simulink model "Quadcopter_v2_full_lqr_BEMT_NEDforwardflight"  (R2021a)
settings: Solver=ode4  StartTime=0.0  StopTime=14  FixedStep=0.001  RelTol=1e-6
values from neighbouring files (symbols this model uses):
  mean_wind = [2.72 , 1.75, .006]    [main_LQR_run.m]
  q = reshape(y(4:7),[4 1])    [deriveLinSys.m]
  r = linspace(floor(nr*0.01)/nr,1,nr)    [main_LQR_run.m]    (also in try1.m = geometry(10,1:nr); try2.m = geometry(10,1:nr))
  x0 = [0,0,0,1,0,0,0,-P.mean_wind,0,0,0]    [main_LQR_run.m]
  xref = [1,1,-8,1,0,0,0,-P.mean_wind]    [main_LQR_run.m]
undefined symbols (not defined in the file or in its folder): HDBK, MIL, Moderate, P
libraries: simulink x1, aerolibwind2 x1
(part 2 of 2)

== matlab function Quadcopter_v2_full_lqr_BEMT_NEDforwardflight/Motor-Rotor_Dynamics/Rotor_Dynamics/correct_thrust2 ==
  data: omega_ideal input; state input; wind input; omega_actual output; P parameter; moments output
function [omega_actual, moments] = fcn(omega_ideal, state,wind, P)
%from "Dynamic Control of Autonomous Quadrotor Flight in an Estimated Wind
%Field," by Sydney, Smyth, and Paley
omega_actual=omega_ideal;

%ensure nonzero rotor speed
if omega_ideal<0
    omega_ideal=0;
end

T_ideal = P.k_t*omega_ideal^2;

phi = state(7);
theta = state(8);
psi = state(9);

%induced velocity of air
v_h = sqrt(T_ideal/(2*P.rho*pi*P.R1^2));

% rotation from inertial frame to body frame
R = [1, 0, 0;0, cos(phi), sin(phi);0, -sin(phi), cos(phi)]*[cos(theta),...
    0, -sin(theta);0, 1, 0;sin(theta), 0, cos(theta)]*[cos(psi),...
    sin(psi), 0;-sin(psi), cos(psi), 0;0, 0, 1];

%find u, v, w (airspeeds on rotor in body frame)
% air_vel = R*(wind - state(4:6));
air_vel = R*(state(4:6)-wind);
% air_vel = R*(state(4:6)+wind);
% air_vel = R*(state(4:6));


%model blade flapping
if sqrt(air_vel(1)^2+air_vel(2)^2)>0.01
    alpha = P.kf_rotor*sqrt(air_vel(1)^2+air_vel(2)^2);
    u_bar = air_vel(1)/sqrt(air_vel(1)^2+air_vel(2)^2);
    v_bar = air_vel(2)/sqrt(air_vel(1)^2+air_vel(2)^2);

    T_flap_vec = T_ideal*[u_bar*sin(alpha), v_bar*sin(alpha), cos(alpha)];
    T_flap = T_flap_vec(3);
else
    T_flap_vec = [0, 0, T_ideal];
    T_flap = T_ideal;
end



if air_vel(3)>2*abs(v_h) 
    
    p = [1 2*air_vel(3) (air_vel(1)^2+air_vel(2)^2+air_vel(3)^2) 0 -v_h^4];
    vi = max(real(roots(p)));

    if norm(air_vel)<=0.5
        vi = v_h;
    end

    T_actual = T_flap*vi/(vi+air_vel(3));
else
    T_actual = T_flap;
end

% omega_actual = sqrt(T_actual/P.k_t);
omega_actual = real(sqrt(complex(T_actual/P.k_t)));

% moments = [0 T_flap_vec(2:-1:1) 0];
moments = [0 0 0 0];

if omega_actual>1000
    omega_actual=1000;
end


end

== matlab function Quadcopter_v2_full_lqr_BEMT_NEDforwardflight/Motor-Rotor_Dynamics/Rotor_Dynamics/correct_thrust3 ==
  data: omega_ideal input; state input; wind input; omega_actual output; P parameter; moments output
function [omega_actual, moments] = fcn(omega_ideal, state,wind, P)
%from "Dynamic Control of Autonomous Quadrotor Flight in an Estimated Wind
%Field," by Sydney, Smyth, and Paley
omega_actual=omega_ideal;

%ensure nonzero rotor speed
if omega_ideal<0
    omega_ideal=0;
end

T_ideal = P.k_t*omega_ideal^2;

phi = state(7);
theta = state(8);
psi = state(9);

%induced velocity of air
v_h = sqrt(T_ideal/(2*P.rho*pi*P.R1^2));

% rotation from inertial frame to body frame
R = [1, 0, 0;0, cos(phi), sin(phi);0, -sin(phi), cos(phi)]*[cos(theta),...
    0, -sin(theta);0, 1, 0;sin(theta), 0, cos(theta)]*[cos(psi),...
    sin(psi), 0;-sin(psi), cos(psi), 0;0, 0, 1];

%find u, v, w (airspeeds on rotor in body frame)
% air_vel = R*(wind - state(4:6));
air_vel = R*(state(4:6)-wind);
% air_vel = R*(state(4:6)+wind);
% air_vel = R*(state(4:6));


%model blade flapping 
if sqrt(air_vel(1)^2+air_vel(2)^2)>0.01
    alpha = P.kf_rotor*sqrt(air_vel(1)^2+air_vel(2)^2);
    u_bar = air_vel(1)/sqrt(air_vel(1)^2+air_vel(2)^2);
    v_bar = air_vel(2)/sqrt(air_vel(1)^2+air_vel(2)^2);

    T_flap_vec = T_ideal*[u_bar*sin(alpha), v_bar*sin(alpha), cos(alpha)];
    T_flap = T_flap_vec(3);
else
    T_flap_vec = [0, 0, T_ideal];
    T_flap = T_ideal;
end



if air_vel(3)>2*abs(v_h)
    
    p = [1 2*air_vel(3) (air_vel(1)^2+air_vel(2)^2+air_vel(3)^2) 0 -v_h^4];
    vi = max(real(roots(p)));

    if norm(air_vel)<=0.5
        vi = v_h;
    end

    T_actual = T_flap*vi/(vi+air_vel(3));
else
    T_actual = T_flap;
end

% omega_actual = sqrt(T_actual/P.k_t);
omega_actual = real(sqrt(complex(T_actual/P.k_t)));

% moments = [0 T_flap_vec(2:-1:1) 0];
moments = [0 0 0 0];

if omega_actual>1000
    omega_actual=1000;
end

end

== matlab function Quadcopter_v2_full_lqr_BEMT_NEDforwardflight/quadcopter/MATLAB Function1 ==
  data: u input; v_rel_b output; wind input; R input
function v_rel_b = body_rel_calcl(u, wind, R)
% v_rel_b: Relative body velocity of quadcopter

wind(3)= -wind(3); %assuming wind from CFD sim is positive upward
v_b = transpose(R)*u  ;
v_rel_b= v_b - transpose(R)*wind; %v = v_rel + v_wind

== matlab function Quadcopter_v2_full_lqr_BEMT_NEDforwardflight/Motor-Rotor_Dynamics/moments_to_motor_speed ==
  data: u input; omega output; P parameter
function omega = fcn(u, P)

omega = u;
%prevent negative F
if u(1)<0
    u(1)=0;
end
%prevent too high of a moment
for i=2:3
    if u(i)>.15*u(1)
        u(i)=.15*u(1);    %why?
    end
end

L = P.L;
k_t = P.k_t;
k_d = P.k_d;

A = [k_t k_t k_t k_t;
    0 -L*k_t 0 L*k_t;
    L*k_t 0 -L*k_t 0;
    -k_d k_d -k_d k_d];
%R matrix just changes which direction the 'front' of the quad is
%without it,quadcopter would be '+' type;with it,quadcopter would be 'x' type
% offset = pi/4;
% R = [1 0 0 0;
%     0 cos(offset) -sin(offset) 0;
%     0 sin(offset) cos(offset) 0;
%     0 0 0 1];
% omega_squared = pinv(A)*R*u; %pinv-Pseudoinverse

omega_squared = pinv(A)*u; %pinv-Pseudoinverse

for i=1:4
    if omega_squared(i) < 0
        omega_squared(i) = 0;
    end
end

omega = sqrt(omega_squared);

== matlab function Quadcopter_v2_full_lqr_BEMT_NEDforwardflight/Motor-Rotor_Dynamics/motor1/control_speed ==
  data: error output; prev_error input; u input; y output; int_u input; desired input; P parameter
function [error, y] = fcn(prev_error, u, int_u, desired, P)

%y = u;
if desired > 5000
    desired = 5000;
end

error = (desired-u);

Ts = P.Ts;

% kd = .2;
% kp = 10;
% ki = 5;

% kd = 0.06;
% kp = 0.1;
% ki = 1;

kd = P.kd_motor;
kp = P.kp_motor;
ki = P.ki_motor;

edot = ((error)-(prev_error))/Ts;

y = (kd*edot + kp*(error) + ki*int_u);

%saturate pwm at 2000
if abs(y) > 2000
    y = sign(y)*2000;
end

== matlab function Quadcopter_v2_full_lqr_BEMT_NEDforwardflight/Motor-Rotor_Dynamics/motor2/control_speed ==
  data: error output; prev_error input; u input; y output; int_u input; desired input; P parameter
function [error, y] = fcn(prev_error, u, int_u, desired, P)

%y = u;
if desired > 5000
    desired = 5000;
end

error = (desired-u);

Ts = P.Ts;

% kd = .2;
% kp = 10;
% ki = 5;

% kd = 0.05;
% kp = 1;
% ki = 1;

kd = P.kd_motor;
kp = P.kp_motor;
ki = P.ki_motor;

edot = ((error)-(prev_error))/Ts;

y = (kd*edot + kp*(error) + ki*int_u);

%saturate pwm at 2000
if abs(y) > 2000
    y = sign(y)*2000;
end

== matlab function Quadcopter_v2_full_lqr_BEMT_NEDforwardflight/Motor-Rotor_Dynamics/motor3/control_speed ==
  data: error output; prev_error input; u input; y output; int_u input; desired input; P parameter
function [error, y] = fcn(prev_error, u, int_u, desired, P)

%y = u;
if desired > 5000
    desired = 5000;
end

error = (desired-u);

Ts = P.Ts;

% kd = .2;
% kp = 10;
% ki = 5;

% kd = 0.05;
% kp = 1;
% ki = 1;

kd = P.kd_motor;
kp = P.kp_motor;
ki = P.ki_motor;

edot = ((error)-(prev_error))/Ts;

y = (kd*edot + kp*(error) + ki*int_u);

%saturate pwm at 2000
if abs(y) > 2000
    y = sign(y)*2000;
end

== matlab function Quadcopter_v2_full_lqr_BEMT_NEDforwardflight/Motor-Rotor_Dynamics/motor4/control_speed ==
  data: error output; prev_error input; u input; y output; int_u input; desired input; P parameter
function [error, y] = fcn(prev_error, u, int_u, desired, P)

%y = u;
if desired > 5000
    desired = 5000;
end

error = (desired-u);

Ts = P.Ts;

% kd = .2;
% kp = 10;
% ki = 5;

% kd = 0.05;
% kp = 1;
% ki = 1;

kd = P.kd_motor;
kp = P.kp_motor;
ki = P.ki_motor;

edot = ((error)-(prev_error))/Ts;

y = (kd*edot + kp*(error) + ki*int_u);

%saturate pwm at 2000
if abs(y) > 2000
    y = sign(y)*2000;
end

== matlab function Quadcopter_v2_full_lqr_BEMT_NEDforwardflight/Motor-Rotor_Dynamics/motor_speed_to_moments ==
  data: u input; F output; P parameter
function F = fcn(u, P)

F = u;

L = P.L;
k_t = P.k_t;
k_d = P.k_d;


A = [k_t k_t k_t k_t;
    0 -L*k_t 0 L*k_t;
    L*k_t 0 -L*k_t 0;
    -k_d k_d -k_d k_d];
%R matrix just changes which direction the 'front' of the quad is
%without it,quadcopter would be '+' type;with it,quadcopter would be 'x' type
% offset = pi/4;
% R = [1 0 0 0;
%     0 cos(offset) -sin(offset) 0;
%     0 sin(offset) cos(offset) 0;
%     0 0 0 1];
% F = R*F;
% F(2:3)=F(3:-1:2);

F = A*u.^2;
end

== matlab function Quadcopter_v2_full_lqr_BEMT_NEDforwardflight/wind/Dryden Wind/Input/DCM//rotation matrix ==
  data: x input; R output
function R = fcn(x)
phi = x(7);theta = x(8);psi = x(9);
% rotation from inertial frame to body frame
R = [1, 0, 0;0, cos(phi), sin(phi);0, -sin(phi), cos(phi)]*[cos(theta),...
    0, -sin(theta);0, 1, 0;sin(theta), 0, cos(theta)]*[cos(psi),...
    sin(psi), 0;-sin(psi), cos(psi), 0;0, 0, 1];
R = inv(R);
end

== matlab function Quadcopter_v2_full_lqr_BEMT_NEDforwardflight/wind/Dryden Wind/Input/MATLAB Function ==
  data: wind input; V output; vel input
function V = fcn(wind,vel)
%#codegen
V = norm(wind - vel);
end

== matlab function Quadcopter_v2_full_lqr_BEMT_NEDforwardflight/wind/Dryden Wind/Input1/DCM//rotation matrix ==
  data: x input; y output
function y = fcn(x)
phi = x(7);theta = x(8);psi = x(9);
% rotation from inertial frame to body frame
R = [1, 0, 0;0, cos(phi), sin(phi);0, -sin(phi), cos(phi)]*[cos(theta),...
    0, -sin(theta);0, 1, 0;sin(theta), 0, cos(theta)]*[cos(psi),...
    sin(psi), 0;-sin(psi), cos(psi), 0;0, 0, 1];
R = inv(R);
y = R;

== matlab function Quadcopter_v2_full_lqr_BEMT_NEDforwardflight/quadcopter/MATLAB Function ==
  settings: updateMethod=DISCRETE
  data: X input; U input; wind input; X_dot output; P parameter; wdot output; R output
function [X_dot,wdot,R]  = quad_model(X,U,wind,P)

%#codegens
%References: Dynamics using Quaternion for full-state feedback control
%adapted from "Onboard State Dependent LQR for Agile Quadrotors"
%see "AIAA paper draft for full model"

%parameters
m = P.m;
g = P.g;
Ix = P.Ix;
Iy = P.Iy;
Iz = P.Iz;
J=[Ix , 0 , 0;
    0 , Iy , 0;
    0 , 0  , Iz];

D   = P.D;
%states
% p_i = X(1:3);
q_i  = X(4:7);
v_i = X(8:10);
w_b = X(11:13);
disp(w_b)


%inputs

F_c = [0;0;U(1)];
tau=[U(2);
     U(3);
     U(4)];
 
%% system dynamics with drag in WORLD FRAME
wind(3)=-wind(3);%wind from CFD data is positive upward
R=quater_rot(q_i);
dp = v_i+wind;
dq = 0.5*quater_mult(q_i)*[0;w_b];
dv = ([0;0;g] - R*F_c-norm(v_i)*R*D*R'*v_i)/m;
dwb = J\(tau-cross(w_b,(J*w_b)));

X_dot=[dp ; dq ; dv ; dwb]';
wdot=dwb;


end


function R = quater_rot(q)

w = q(1);
x = q(2);
y = q(3);
z = q(4);

Q = [w -x -y -z;...
     x w -z y;...
     y z w -x;...
     z -y x w];

Qc =[w -x -y -z;...
     x w z -y;...
     y -z w x;...
     z y -x w];
t = Qc'*Q;
R = t(2:4,2:4);
end


function Q = quater_mult(q)

w = q(1);
x = q(2);
y = q(3);
z = q(4);

Q = [w -x -y -z;...
     x w -z y;...
     y z w -x;...
     z -y x w];

end

== matlab function Quadcopter_v2_full_lqr_BEMT_NEDforwardflight/wind/Dryden Wind/Input1/MATLAB Function ==
  data: wind input; V output; vel input; P parameter
function V = fcn(wind,vel,P)
%#codegen
V = norm(wind - vel);
end

== matlab function Quadcopter_v2_full_lqr_BEMT_NEDforwardflight/wind/Dryden Wind/Select velocities/Merge Subsystems/convert to inertial frame ==
  data: ug input; ugw output; vg input; wg input; dcm input; vgw output; wgw output
function [ugw,vgw,wgw] = fcn(ug,vg,wg,dcm)
%#codegen
u = dcm*[ug;vg;wg];
ugw = u(1);
vgw = u(2);
wgw = u(3);

== matlab function Quadcopter_v2_full_lqr_BEMT_NEDforwardflight/Controller /High Level Controller/trajectory/MATLAB Function ==
  data: t input; xdes output; P parameter
function xdes = getref(t,P)

% This function tracks time and match nominal trajectory at next nearest
% time
% Input:
% nomTraj is the nominal trajectory with t
% 
nomTraj = P.nomTraj;
idxA = find(nomTraj(:,1)>=t);
idx=idxA(1);
xdes=nomTraj(idx,2:end);

== matlab function Quadcopter_v2_full_lqr_BEMT_NEDforwardflight/MATLAB Function ==
  data: u input; omega output; P parameter
function omega = motor_omega(u, P)

%omega = u;
%prevent negative F because the calculation only need the value of fc
% if u(1)<0
%     u(1)=-u(1);
% end
%prevent too high of a moment
for i=2:3
    if u(i)>.15*u(1)
        u(i)=.15*u(1);    %why?
    end
end

L = P.l;
b= P.b;
k = P.k;
% 
A = [b b b b;
    0 L*b 0 -L*b;
    L*b 0 -L*b 0;   %from BMET Code 
    k -k k -k];  %

% A = [b b b b;
%     0 -L*b 0 L*b;
%     -L*b 0 L*b 0;   %from source Trajectory tracking control design with command-filtered compensation for a quadrotor
%     -k k -k k]; 


% A = [b b b b;
%     0 -L*b 0 L*b;
%     L*b 0 -L*b 0;   %Tryng my ways
%     k -k k -k];  %

%R matrix just changes which direction the 'front' of the quad is
%without it,quadcopter would be '+' type;with it,quadcopter would be 'x' type
% offset = pi/4;
% R = [1 0 0 0;
%     0 cos(offset) -sin(offset) 0;
%     0 sin(offset) cos(offset) 0;
%     0 0 0 1];
% omega_squared = pinv(A)*R*u; %pinv-Pseudoinverse

omega_squared = pinv(A)*u'; %pinv-Pseudoinverse

for i=1:4
    if omega_squared(i) < 0
%         omega_squared(i) = 0;
        omega_squared(i)=abs(omega_squared(i));
    end
end

omega = sqrt(omega_squared);

== matlab function Quadcopter_v2_full_lqr_BEMT_NEDforwardflight/sensors/GPS ==
  settings: updateMethod=DISCRETE
  data: x input; GPS output; P parameter
function GPS  = fcn(x,P)
%#codegen
Pn = x(1);
Pe = x(2);
Pd = x(3);

%% model1 
bias_gps_x=P.bias_gps_x;
bias_gps_y=P.bias_gps_y;
bias_gps_z=P.bias_gps_z;
sigma_gps=P.sigma_gps;
Pn = Pn + bias_gps_x + sigma_gps*randn;
Pe = Pe + bias_gps_y + sigma_gps*randn;
Pd = Pd + bias_gps_z + sigma_gps*randn;
GPS=[Pn;Pe;Pd];
%% model2
%     % GPS parameters
%     Ts_gps = 1; % sample rate of GPS in s
%     beta_gps = 1/1100; % 1/s
%     sigma_n_gps = 0.21;
%     sigma_e_gps = 0.21; 
%     sigma_h_gps = 0.40;
%     % persistent variables that define random walk of GPS sensors
%     persistent eta_n;
%     persistent eta_e;
%     persistent eta_h;
%     
%     
%     if t==0  % initialize persistent variables
%         eta_n = 0;
%         eta_e = 0;
%         eta_h = 0;
%     else      % propagate persistent variables
%         eta_n = exp(beta_gps*Ts_gps)*eta_n + sigma_n_gps*randn;
%         eta_e = exp(beta_gps*Ts_gps)*eta_e + sigma_e_gps*randn;
%         eta_h = exp(beta_gps*Ts_gps)*eta_h + sigma_h_gps*randn;
%     end
%     
%     % construct North, East, and altitude GPS measurements
%     y_gps_n = Pn + eta_n;
%     y_gps_e = Pe + eta_e; 
%     y_gps_h = Pd + eta_h; 
%     
%     GPS=[y_gps_n;y_gps_e;y_gps_h];

end

== matlab function Quadcopter_v2_full_lqr_BEMT_NEDforwardflight/wind/sinusoidal_wind/sinusoidal part ==
  data: LES input; y output; t input
function y = fcn(LES,t)
ux=2.7;
uy=1.7;
uz=0;
dx = LES(1) - ux + 3*sin(2*pi*(1/50)*t); 
dy = LES(2) - uy + 2*sin(2*pi*(1/50)*t); 
dz = LES(3) - uz + 0.5*sin(2*pi*(1/50)*t); 
y = [dx;dy;dz];

== matlab function Quadcopter_v2_full_lqr_BEMT_NEDforwardflight/quadcopter/initial states/MATLAB Function1 ==
  data: X0 output
function X0  = fcn()
% X0 = [10*randn;10*randn;10*randn;2*randn;2*randn;2*randn;...
%      (pi/4)*randn;(pi/4)*randn;(pi/4)*randn;0;0;0;];
X0 = [10*randn;10*randn;10*randn;1*randn;1*randn;1*randn;...
     0.1*randn;0.1*randn;0.1*randn;0.1*randn;0.1*randn;0.1*randn];
end

== matlab function Quadcopter_v2_full_lqr_BEMT_NEDforwardflight/sensors/sensors ==
  settings: updateMethod=DISCRETE
  data: x input; x_dot input; P parameter; Accel_Gyro output; B_b output
function [Accel_Gyro,B_b] = fcn(x,x_dot,P)
%#codegen
Pn = x(1);
Pe = x(2);
Pd = x(3);
Pn_dot = x(4);Pn_ddot = x_dot(4);
Pe_dot = x(5);Pe_ddot = x_dot(5);
Pd_dot = x(6);Pd_ddot = x_dot(6);
phi = x(7);
theta = x(8);
psi = x(9);
p = x(10);
q = x(11);
r = x(12);

g = P.g ;

bias_gyro_x=P.bias_gyro_x;
bias_gyro_y=P.bias_gyro_y;
bias_gyro_z=P.bias_gyro_z;
sigma_gyro =P.sigma_gyro;

bias_accel_x = P.bias_accel_x;
bias_accel_y = P.bias_accel_y;
bias_accel_z = P.bias_accel_z;
sigma_accel = P.sigma_accel;

bias_B_x = P.bias_B_x;
bias_B_y = P.bias_B_y;
bias_B_z = P.bias_B_z;
sigma_B = P.sigma_B;
% simulate rate gyros (units are rad/sec)
y_gyro_x = p + bias_gyro_x + sigma_gyro*randn;
y_gyro_y = q + bias_gyro_y + sigma_gyro*randn;
y_gyro_z = r + bias_gyro_z + sigma_gyro*randn;

% simulate accelerometers (units of g)
Pd_ddot = Pd_ddot- g;
P_ddot=[Pn_ddot;Pe_ddot;Pd_ddot];
%rotation matrix which can rotate the vector from inertial frame to body
%frame
Rbi=[                          cos(theta)*cos(psi)                            cos(theta)*sin(psi)         -sin(theta);
    sin(phi)*sin(theta)*cos(psi)-cos(phi)*sin(psi) sin(phi)*sin(theta)*sin(psi)+cos(phi)*cos(psi) sin(phi)*cos(theta);
    cos(phi)*sin(theta)*cos(psi)+sin(phi)*sin(psi) cos(phi)*sin(theta)*sin(psi)-sin(phi)*cos(psi) cos(phi)*cos(theta)];

a=Rbi*P_ddot;
ax=a(1);ay=a(2);az=a(3);
y_accel_x = ax + bias_accel_x + sigma_accel*randn;
y_accel_y = ay + bias_accel_y + sigma_accel*randn;
y_accel_z = az + bias_accel_z + sigma_accel*randn;

Accel_Gyro =[y_accel_x;
             y_accel_y;
             y_accel_z;
             y_gyro_x;
             y_gyro_y;
             y_gyro_z;];

%simulate the Magnetometer sensor
% B_i=[1/sqrt(2);0;1/sqrt(2)];
B_i = P.B_i;

B_b=Rbi*B_i;
B_b(1) = B_b(1) + bias_B_x + sigma_B*randn;
B_b(2) = B_b(2) + bias_B_y + sigma_B*randn;
B_b(3) = B_b(3) + bias_B_z + sigma_B*randn;
end

== matlab function Quadcopter_v2_full_lqr_BEMT_NEDforwardflight/BEMT/BEMT Adjustment ==
  settings: updateMethod=DISCRETE
  data: rpm_guesses input; RPM output; V_rel_b input; P parameter; RPM2 output; Tau_initial output; Tau_final output; power output; T_final output; U_final output; geometry data_store_memory; local_param output
function [RPM,RPM2,Tau_initial,Tau_final,power,T_final,U_final,local_param] = FWF(rpm_guesses,V_rel_b, P)


% governing equations
% governing equations

% T=T1+T2+T3+T4 ;
% TA1=l*(T4-T2) ;   roll positive right wing down
% TA2=l*(T1-T3) ;   pitch up positive
% TA3=ta1+ta2+ta3+ta4 ;

% it looks like in atitude control output of the functin should be pitch
% down positive
% Not Related with LQR CONTROL ASMA*

%%
% predefining vriables for Codegen

k = P.k;
b = P.b;
l = P.l;
T_final=0;
Tau_initial=zeros(3,1);
Tau_final=zeros(3,1);
T2=zeros(4,1);
pow=zeros(4,1);

TA=zeros(3,1);
TA1=zeros(4,1);
TA2=zeros(4,1);
TA3=zeros(4,1);
ta1=zeros(4,1);
ta2=zeros(4,1);
ta3=zeros(4,1);

RPM2=single(zeros(4,1));
RPM=zeros(4,1);

T = b * rpm_guesses.^2;       % requested thrust from rotor r
Tau = k * rpm_guesses.^2;     % requested torques from rotor r

for i=1:4
    % optimization to find optimum rpm where both momentum annd blade element theories match
    
    subfcn2 = @(rpm) try1(rpm,V_rel_b,T(i));
    
    rpm=golden_search(0,25000,subfcn2); %limits of RPM, checked that the higher limit goes beyond 25000 so chaging from 100 16000
    
    [~,roll,pitch,yaw]=try1(rpm,V_rel_b,T(i));
    
    % rpm to rad/second
    RPM(i)=rpm ;%*2*pi/60; NO NEED ASMA
    
    % torques of a rotor - rotor 1 is the leading edge rotor,left
    % number 2, right number 4, aft number, 1 and 3 ccw. 2 and 4 cw.
    
    heading=atan(V_rel_b(2)/(V_rel_b(1)+0.000001));
    ta1(i) = roll * cos(heading) * (-1)^(i+1) - pitch * sin(heading);
    ta2(i) = roll * sin(heading) * (-1)^(i+1) + pitch * cos(heading) ;
    % the sign will be taken care of in Matrix M -- no worries!
    ta3(i) = yaw * (+1)^(i+1); %??? ASMA
    
end

Tau_initial=[sum(ta1);sum(ta2);sum(ta3)];

%% new addition to help with yaw moment

% here we need to find a way to change RPMs a bit such that they also
% provide the required Ta3. So, we can find the thrust and torque
% coefficients for a specific time and flight condition.

bb=T./RPM.^2;
kk=ta3./RPM.^2;

M=[bb'; ...
  0,bb(2)*l,0,-bb(4)*l;...
  bb(1)*l,0,-bb(3)*l,0;...
  kk(1),-kk(2),kk(3),-kk(4)];

% M=double([bb'; ...
%   0,-bb(2)*l,0,bb(4)*l;...
%   bb(1)*l,0,-bb(3),0;...
%   kk(1),-kk(2),kk(3),-kk(4)]);  %ASMA

T_tot=sum(T);

% we use the requsted thrust and torque - here we used the actual
% conventions, down pos z, right wing pos y, pointing to nose pos x
TA(1) = l* (T(2)-T(4)) - Tau_initial(1); % roll
TA(2) = l* (T(1)-T(3)) - Tau_initial(2); % pitch
TA(3) = dot([k,-k,k,-k],rpm_guesses.^2'); % yaw



%ASMA
%  TA(1) = l* (T(4)-T(2)) - Tau_initial(1); % roll
% TA(2) = l* (T(1)-T(3)) - Tau_initial(2); % pitch
% TA(3) = dot([-k,k,-k,k],rpm_guesses.^2'); % yaw

u_temp= [T_tot;TA(1);TA(2);TA(3)];
% newly obtained RPMs Original
% RPM2=(M\[T_tot;TA(1);TA(2);TA(3)]).^0.5;

%%ADDED BY ASMA
RPM_SQ = pinv(M)*u_temp;

for i=1:4
    if RPM_SQ(i) < 0
        RPM_SQ(i) = 0;
    end
end

RPM2 = sqrt(RPM_SQ);

% now let's see how much thrust and torque they make

for i=1:4
    % input to propeller code must be RPM not rev/sec
    
    subfcn2 = @(T) try2(T,rpm,V_rel_b);
    
    T=golden_search(0,40,subfcn2);  %THIS IS FOR THURST
    
    [~,roll,pitch,yaw,T]=try2(T,RPM2(i),V_rel_b);
    pow(i)=yaw * RPM2(i);
    T2(i)=T;
    heading=atan(V_rel_b(2)/(V_rel_b(1)+0.000001));
    TA1(i) = roll * cos(heading) * (-1)^(i+1) - pitch * sin(heading);
    TA2(i) = roll * sin(heading) * (-1)^(i+1) + pitch * cos(heading) ;
    TA3(i)=yaw* (-1)^(i+1);
end

TA_rotor=[sum(TA1);sum(TA2);sum(TA3)];

% here since we don't use negative thrusts, conventions are changed
T_final=sum(T2);
Tau_final(1,1)=l*(T2(2)-T2(4))+TA_rotor(1) ; % roll
Tau_final(2,1)=l*(T2(1)-T2(3))+ TA_rotor(2) ; % pitch
Tau_final(3,1)=TA_rotor(3) ;

%ASMA
%  Tau_final(1,1)=l*(T2(4)-T2(2))+ TA_rotor(1) ; % roll 

power = sum(pow) ;

U_final=[T_final,Tau_final'];
local_param= [bb , kk];
end
